simulink model "Proportional_Controller_Model"  (R2021a)
settings: Solver=VariableStepAuto  StartTime=0.0  StopTime=ExpPeriod  RelTol=1e-3
values from neighbouring files (symbols this model uses):
  Kp = 2.2    [Control_Kp.m]    (also in Control_PI.m)
  Ts = 0.02    [Control_Kp.m]    (also in Control_PI.m; Identification.m; Model_Verification.m)
undefined symbols (not defined in the file or in its folder): sigbuilder_block
settings Model: Creator=moesaab  LastModifiedBy=moesaab

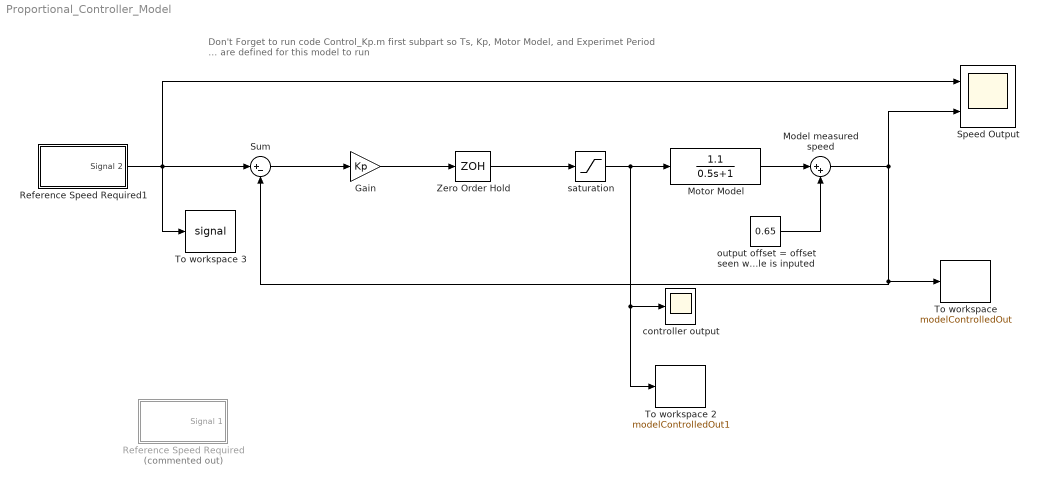
== system Proportional_Controller_Model ==
  note: Don't Forget to run code Control_Kp.m first subpart so Ts, Kp, Motor Model, and Experimet Period ... are defined for this model to run
  "\tTo workspace 2" : ToWorkspace  VariableName=modelControlledOut1  SampleTime=Ts
      settings: Save2DSignal=2-D array (concatenate along first dimension)
  Gain : Gain  Gain=Kp
  Model measured speed : Sum  Inputs=|++
  Motor Model : TransferFcn  Numerator=1.1  Denominator=[0.5 1]
  Reference Speed Required : Subsystem  Tag=STV Subsys  Commented=on  LoadFcn=sigbuilder_block('load');  StartFcn=sigbuilder_block('start');  StopFcn=sigbuilder_block('stop');  ClipboardFcn=sigbuilder_block('clipboard');  mask(Sigbuilder block){tuvar=[0:10]}
      mask help: Simulink:masks:SigbuilderBlock_MD
      mask init:
      | if ~strcmp(get_param(bdroot(gcbh),'SimulationStatus'),'stopped') tuvar = sigbuilder_block('maskInit'); end
      settings: CopyFcn=sigbuilder_block('copy');  DeleteFcn=sigbuilder_block('delete');  ModelCloseFcn=sigbuilder_block('modelClose');  PreSaveFcn=sigbuilder_block('preSave');  PauseFcn=sigbuilder_block('pause');  ContinueFcn=sigbuilder_block('continue');  NameChangeFcn=sigbuilder_block('namechange');  OpenFcn=sigbuilder_block('open',[69.8614 59.8812 1221.86 496.158 ]);  CloseFcn=sigbuilder_block('close');
      mask Display: plot(0, 0, 100, 100,[2, 2, 32, 32, 2], [68, 8, 8, 68, 68],[32, 2], [38, 38], [32, 19, 2],[53, 60, 44], [32, 17, 17, 2],[16, 16, 31, 31]);txt = getActiveGroup(gcbh);text(2, 100, txt,'verticalAlignment', 'top');
  Reference Speed Required1 : Subsystem  Tag=STV Subsys  LoadFcn=sigbuilder_block('load');  StartFcn=sigbuilder_block('start');  StopFcn=sigbuilder_block('stop');  ClipboardFcn=sigbuilder_block('clipboard');  mask(Sigbuilder block){tuvar=[0:10]}
      mask help: Simulink:masks:SigbuilderBlock_MD
      mask init:
      | if ~strcmp(get_param(bdroot(gcbh),'SimulationStatus'),'stopped') tuvar = sigbuilder_block('maskInit'); end
      settings: CopyFcn=sigbuilder_block('copy');  DeleteFcn=sigbuilder_block('delete');  ModelCloseFcn=sigbuilder_block('modelClose');  PreSaveFcn=sigbuilder_block('preSave');  PauseFcn=sigbuilder_block('pause');  ContinueFcn=sigbuilder_block('continue');  NameChangeFcn=sigbuilder_block('namechange');  OpenFcn=sigbuilder_block('open',[69.8614 59.8812 1221.86 496.158 ]);  CloseFcn=sigbuilder_block('close');
      mask Display: plot(0, 0, 100, 100,[2, 2, 32, 32, 2], [68, 8, 8, 68, 68],[32, 2], [38, 38], [32, 19, 2],[53, 60, 44], [32, 17, 17, 2],[16, 16, 31, 31]);txt = getActiveGroup(gcbh);text(2, 100, txt,'verticalAlignment', 'top');
  Speed Output : Scope  NumInputPorts=2
  Sum : Sum  Inputs=|+-
  To workspace : ToWorkspace  VariableName=modelControlledOut  SampleTime=Ts
      settings: Save2DSignal=2-D array (concatenate along first dimension)
  To workspace 3 : ToWorkspace  VariableName=signal  SampleTime=Ts
      settings: Save2DSignal=2-D array (concatenate along first dimension)
  Zero Order Hold : ZeroOrderHold  SampleTime=-1
  "controller output " : Scope
  output offset = offset seen when input offset 0.3 duty cycle is inputed : Constant  Value=0.65
  saturation : Saturate  LowerLimit=0
  wires:
  Sum/1 -> Gain/1
  output offset = offset seen when input offset 0.3 duty cycle is inputed/1 -> Model measured speed/2
  Gain/1 -> Zero Order Hold/1
  saturation/1 -> Motor Model/1, "\tTo workspace 2"/1, "controller output "/1
  Reference Speed Required1/1(Signal 2) -> Speed Output/1, To workspace 3/1, Sum/1
  Motor Model/1 -> Model measured speed/1
  Model measured speed/1 -> Sum/2, To workspace/1, Speed Output/2
  Zero Order Hold/1 -> saturation/1

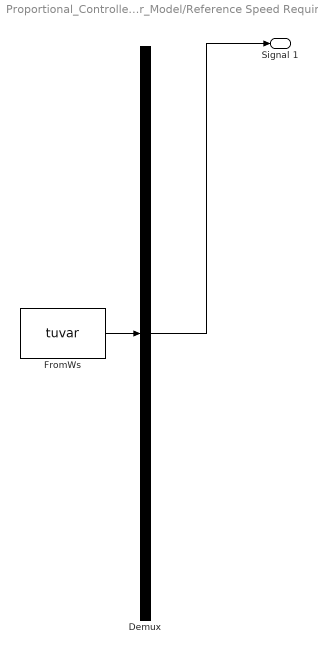
== system Proportional_Controller_Model/Reference Speed Required ==
  Demux : Demux  Tag=STV Demux  Outputs=1
      settings: DisplayOption=none
  FromWs : FromWorkspace  Tag=STV FromWs  VariableName=tuvar  SampleTime=Ts
      SigBuilderData=|
      | common.afterFinalStr = 'Extrapolate'
      | common.sampleTime = 'Ts'
      | dataSet.timeRange = [0 50]
      | dataSet.name = 'Group 1'
      | sbobj.Groups.Name = 'Group 1'
      | sbobj.Groups.Signals.Name = 'Signal 1'
      | sbobj.Groups.Signals.XData = [0 6.3 6.3 10.1 10.1 15.25 15.25 18.05 18.05 22.1 22.1 29.8 29.8 35.1 35.1 39.7 39.7 50]
      | sbobj.Groups.Signals.YData = [0.698 0.698 0.899 0.899 1.001 1.001 0.798 0.798 0.721 0.721 0.898359090909 0.898534090909 1.129 1.129 1.002 1.002 0.942 0.942]
      | sbobj.Groups.TimeRange = [0 50]
  Signal 1 : Outport  Tag=STV Outport
  wires:
  Demux/1 -> Signal 1/1
  FromWs/1 -> Demux/1

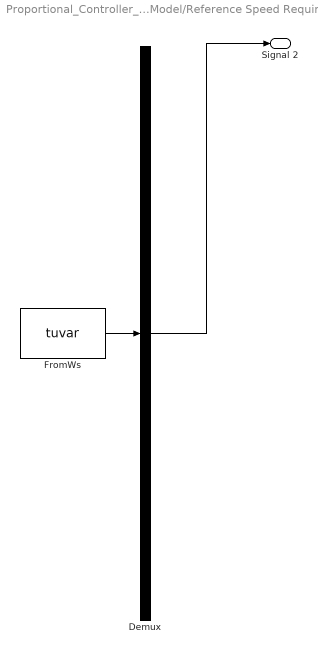
== system Proportional_Controller_Model/Reference Speed Required1 ==
  Demux : Demux  Tag=STV Demux  Outputs=1
      settings: DisplayOption=none
  FromWs : FromWorkspace  Tag=STV FromWs  VariableName=tuvar  SampleTime=Ts
      SigBuilderData=|
      | common.afterFinalStr = 'Extrapolate'
      | common.sampleTime = 'Ts'
      | dataSet.timeRange = [0 50]
      | dataSet.name = 'Group 1'
      | sbobj.Groups.Name = 'Group 1'
      | sbobj.Groups.Signals.Name = 'Signal 2'
      | sbobj.Groups.Signals.XData = [0 5 5 10 10 15 15 20 20 22.1 25.45 29.8 29.8 35.1 35.1 39.95 39.95 44.95 44.95 50]
      | sbobj.Groups.Signals.YData = [0.698 0.698 0.802 0.802 0.9 0.9 1.002 1.002 1.1 1.1 1.10087012987 1.102 1.198 1.198 1.1 1.1 1.002 1.002 0.902 0.902]
      | sbobj.Groups.TimeRange = [0 50]
  Signal 2 : Outport  Tag=STV Outport
  wires:
  Demux/1 -> Signal 2/1
  FromWs/1 -> Demux/1
